simulink model "Kinematic_control_path_tracking"  (R2022b)
settings: Solver=VariableStepAuto  StartTime=0.0  StopTime=T_final*2  RelTol=1e-3
values from neighbouring files (symbols this model uses):
  d = 0.1    [Run_model.m]
  kx = 4    [Run_model.m]
  ky = 4    [Run_model.m]
  R = 1e-5    (= 1e-05)    [Run_model.m]
  Ts = 0.01    [Run_model.m]    (also in imu.m)
  u0 = [0;0]    [Run_model.m]
  z_initial = [theta0;x0;y0]    [Run_model.m]
libraries: simulink x1, sharedTrackingLibrary x1
settings Model: Creator=Abelb  LastModifiedBy=RASLab-Distributed

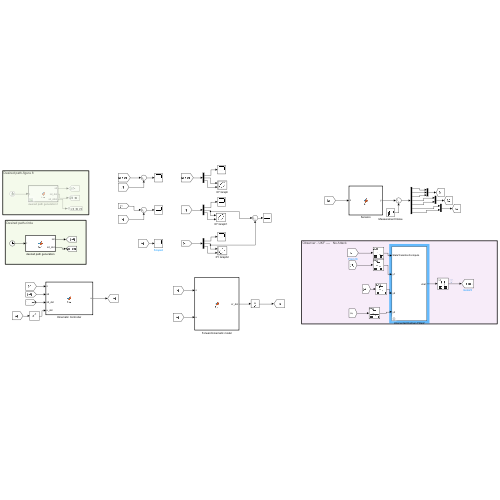
[thumbnail: Simulink's stored preview of the top-level diagram]
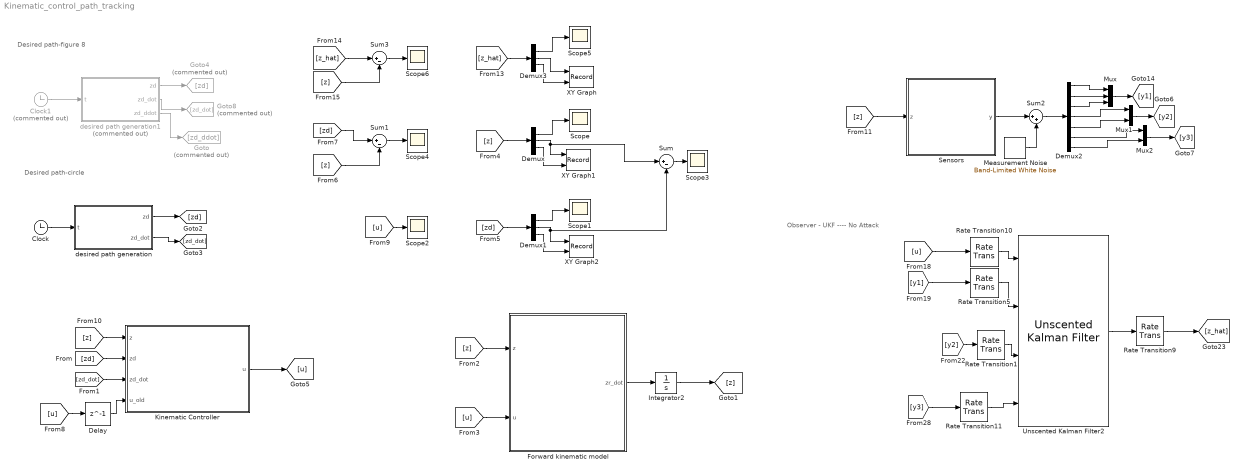
== system Kinematic_control_path_tracking ==
  note: Desired path-circle
  note: Desired path-figure 8
  note: Observer - UKF ---- No Attack
  Clock : Clock
  Clock1 : Clock  Commented=on
  Delay : Delay  DelayLength=1  InitialCondition=u0
  Demux : Demux  Outputs=3
  Demux1 : Demux  Outputs=3
  Demux2 : Demux  Outputs=n_meas
  Demux3 : Demux  Outputs=3
  Forward kinematic model : MATLAB Function  TreatAsAtomicUnit=on
  Goto : Goto  Commented=on  GotoTag=zd_ddot
  Goto4 : Goto  Commented=on  GotoTag=zd
  Goto8 : Goto  Commented=on  GotoTag=zd_dot
  Integrator2 : Integrator  InitialCondition=z_initial
  Kinematic Controller : MATLAB Function  TreatAsAtomicUnit=on
  Measurement Noise : simulink/Sources/Band-Limited White Noise  Cov=R*Ts  Ts=Ts  seed=[23341]
  Mux : Mux  Inputs=3
  Mux1 : Mux  Inputs=2
  Mux2 : Mux  Inputs=2
  Rate Transition1 : RateTransition  InitialCondition=[0 0]  OutPortSampleTime=Ts
  Rate Transition10 : RateTransition  InitialCondition=[0 0]  OutPortSampleTime=Ts
  Rate Transition11 : RateTransition  InitialCondition=[0 0]  OutPortSampleTime=Ts
  Rate Transition5 : RateTransition  InitialCondition=[0 0 0]  OutPortSampleTime=Ts
  Rate Transition9 : RateTransition  Integrity=off  InitialCondition=1.6  OutPortSampleTime=0
  Scope{,1..6} (7 alike) : Scope
  Sensors : MATLAB Function  TreatAsAtomicUnit=on
  Sum : Sum  Inputs=|+-
  Sum1 : Sum  Inputs=|+-
  Sum2 : Sum  Inputs=|++
  Sum3 : Sum  Inputs=|+-
  Unscented Kalman Filter2 : sharedTrackingLibrary/Unscented Kalman Filter  StateTransitionFcn=Dynamicfcn  HasAdditiveProcessNoise=Additive  ProcessNoise=diag([1 1 1])  HasTimeVaryingProcessNoise=off  HasStateTransitionFcnExtraArgument=1  InitialState=z_hat0  InitialStateCovariance=0.1  Alpha=1e-2  Beta=2  Kappa=0  MeasurementFcn1=imu  HasMeasurementEnablePort1=off  HasAdditiveMeasurementNoise1=Additive  MeasurementNoise1=diag([R R R])  HasTimeVaryingMeasurementNoise1=off  HasMeasurementFcnExtraArgument1=0  HasMeasurementWrapping1=off  MeasurementFcn2=encoder  HasMeasurementEnablePort2=off  HasAdditiveMeasurementNoise2=Additive  MeasurementNoise2=diag([R R])  HasTimeVaryingMeasurementNoise2=off  HasMeasurementFcnExtraArgument2=0  HasMeasurementWrapping2=off  MeasurementFcn3=gps  HasMeasurementEnablePort3=off  HasAdditiveMeasurementNoise3=Additive  MeasurementNoise3=diag([R R])  HasTimeVaryingMeasurementNoise3=off  HasMeasurementFcnExtraArgument3=0  HasMeasurementWrapping3=off  MeasurementFcn4=mfcn3  HasMeasurementEnablePort4=off  HasAdditiveMeasurementNoise4=Additive  MeasurementNoise4=R  HasTimeVaryingMeasurementNoise4=off  HasMeasurementFcnExtraArgument4=0  HasMeasurementWrapping4=off  MeasurementFcn5=myMeasurementFcn  HasMeasurementEnablePort5=off  HasAdditiveMeasurementNoise5=Additive  MeasurementNoise5=1  HasTimeVaryingMeasurementNoise5=off  HasMeasurementFcnExtraArgument5=0  HasMeasurementWrapping5=off  EnableMultirate=off  StateTransitionFcnSampleTime=1  MeasurementFcn1SampleTime=1  MeasurementFcn2SampleTime=1  MeasurementFcn3SampleTime=1  MeasurementFcn4SampleTime=1  MeasurementFcn5SampleTime=1  UseCurrentEstimator=off  OutputStateCovariance=off  DataType=double  SampleTime=Ts  NumberOfMeasurements=3
  XY Graph : Record  FileSettingsInternal="{\"entries\":[{\"content\":{\"excelSettings\":{\"content\":{},\"type\":\"Streamout.ExcelSettings\"}},\"type\":\"Streamout.FileSettingStorage\",\"uuid\":\"53b03b39-55e0-4fa9-afe4-2bd9ebb48c30\"}],\"packageUris\":[\"http://schema.mathworks.com/mf0/streamout_blocks/R2020a\"],\"version\":\"1.0\"}"  Layout=[1 1]  SignalsInternal="{\"entries\":[{\"content\":{\"signals\":[{\"content\":{\"blockPath\":[\"Kinematic_control_path_tracking/XY Graph\"],\"channel\":[],\"dimensions\":[1],\"domain\":\"Kinematic_control_path_tracking/XY Graph\",\"lineColor\":\"#a2142f\",\"plots\":[1],\"port\":1,\"sid\":[\"\"],\"signalID\":23982,\"signalName\":\"Demux3:2\"},\"type\":\"RecordBlkView.Signal\",\"uuid\":\"5156a42c-5bae-4aca-bacc-39f4cef39f7f\"},{\"content\":{\"blockPath\":[\"Kinematic_control_path_tracking/XY Graph\"],\"channel\":[],\"dimensions\":[1],\"domain\":\"Kinematic_control_path_tracking/XY Graph\",\"lineColor\":\"#139fff\",\"plots\":[1],\"port\":2,\"sid\":[\"\"],\"signalID\":23986,\"signalName\":\"Demux3:3\"},\"type\":\"RecordBlkView.Signal\",\"uuid\":\"2cf1826c-70a3-4cdb-a73e-eee623f68542\"}]},\"type\":\"RecordBlkView.InputSignals\",\"uuid\":\"c4e639f7-235e-4a76-b281-eb1d9f92212a\"}],\"packageUris\":[\"http://schema.mathworks.com/mf0/streamout_blocks/R2020a\"],\"version\":\"1.0\"}"  VisualizationBindings="{\"xyplotplugin\":{\"info\":[{\"series\":[{\"bindingParametersList\":[{\"parameter\":\"X-Axis\",\"signalID\":23982,\"signalName\":\"Demux3:2\"},{\"parameter\":\"Y-Axis\",\"signalID\":23986,\"signalName\":\"Demux3:3\"}],\"seriesID\":42700}],\"subplotID\":1}]}}"  CompatibilityTag=XY
  XY Graph1 : Record  FileSettingsInternal="{\"entries\":[{\"content\":{\"excelSettings\":{\"content\":{},\"type\":\"Streamout.ExcelSettings\"}},\"type\":\"Streamout.FileSettingStorage\",\"uuid\":\"22695cf6-89d7-43ca-b8cc-e55b69a454ec\"}],\"packageUris\":[\"http://schema.mathworks.com/mf0/streamout_blocks/R2020a\"],\"version\":\"1.0\"}"  Layout=[1 1]  SignalsInternal="{\"entries\":[{\"content\":{\"signals\":[{\"content\":{\"blockPath\":[\"Kinematic_control_path_tracking/XY Graph1\"],\"channel\":[],\"dimensions\":[1],\"domain\":\"Kinematic_control_path_tracking/XY Graph1\",\"lineColor\":\"#a2142f\",\"plots\":[1],\"port\":1,\"sid\":[\"\"],\"signalID\":23990,\"signalName\":\"Demux:2\"},\"type\":\"RecordBlkView.Signal\",\"uuid\":\"5f30c967-a085-4e3c-978a-3d45b454423d\"},{\"content\":{\"blockPath\":[\"Kinematic_control_path_tracking/XY Graph1\"],\"channel\":[],\"dimensions\":[1],\"domain\":\"Kinematic_control_path_tracking/XY Graph1\",\"lineColor\":\"#139fff\",\"plots\":[1],\"port\":2,\"sid\":[\"\"],\"signalID\":23994,\"signalName\":\"Demux:3\"},\"type\":\"RecordBlkView.Signal\",\"uuid\":\"e37d4cd6-5af5-4e48-88eb-1684f785dfd2\"}]},\"type\":\"RecordBlkView.InputSignals\",\"uuid\":\"b7753eae-dfa1-472a-a4ee-c8d1f4983262\"}],\"packageUris\":[\"http://schema.mathworks.com/mf0/streamout_blocks/R2020a\"],\"version\":\"1.0\"}"  VisualizationBindings="{\"xyplotplugin\":{\"info\":[{\"series\":[{\"bindingParametersList\":[{\"parameter\":\"X-Axis\",\"signalID\":23990,\"signalName\":\"Demux:2\"},{\"parameter\":\"Y-Axis\",\"signalID\":23994,\"signalName\":\"Demux:3\"}],\"seriesID\":7810}],\"subplotID\":1}]}}"  CompatibilityTag=XY
  XY Graph2 : Record  FileSettingsInternal="{\"entries\":[{\"content\":{\"excelSettings\":{\"content\":{},\"type\":\"Streamout.ExcelSettings\"}},\"type\":\"Streamout.FileSettingStorage\",\"uuid\":\"eace55e5-3c6d-4366-b246-c90901abd758\"}],\"packageUris\":[\"http://schema.mathworks.com/mf0/streamout_blocks/R2020a\"],\"version\":\"1.0\"}"  Layout=[1 1]  SignalsInternal="{\"entries\":[{\"content\":{\"signals\":[{\"content\":{\"blockPath\":[\"Kinematic_control_path_tracking/XY Graph2\"],\"channel\":[],\"dimensions\":[1],\"domain\":\"Kinematic_control_path_tracking/XY Graph2\",\"lineColor\":\"#a2142f\",\"plots\":[1],\"port\":1,\"sid\":[\"\"],\"signalID\":23998,\"signalName\":\"Demux1:2\"},\"type\":\"RecordBlkView.Signal\",\"uuid\":\"c09d6a8b-b75d-4225-bd49-b55b8471079b\"},{\"content\":{\"blockPath\":[\"Kinematic_control_path_tracking/XY Graph2\"],\"channel\":[],\"dimensions\":[1],\"domain\":\"Kinematic_control_path_tracking/XY Graph2\",\"lineColor\":\"#139fff\",\"plots\":[1],\"port\":2,\"sid\":[\"\"],\"signalID\":24002,\"signalName\":\"Demux1:3\"},\"type\":\"RecordBlkView.Signal\",\"uuid\":\"1f0564bc-c8d1-4d71-ab9b-9d1cb6ef22b8\"}]},\"type\":\"RecordBlkView.InputSignals\",\"uuid\":\"f5b7b8dd-13dd-4d16-8a9c-72a61d8133b0\"}],\"packageUris\":[\"http://schema.mathworks.com/mf0/streamout_blocks/R2020a\"],\"version\":\"1.0\"}"  VisualizationBindings="{\"xyplotplugin\":{\"info\":[{\"series\":[{\"bindingParametersList\":[{\"parameter\":\"X-Axis\",\"signalID\":23998,\"signalName\":\"Demux1:2\"},{\"parameter\":\"Y-Axis\",\"signalID\":24002,\"signalName\":\"Demux1:3\"}],\"seriesID\":9465}],\"subplotID\":1}]}}"  CompatibilityTag=XY
  desired path generation : MATLAB Function  TreatAsAtomicUnit=on
  desired path generation1 : MATLAB Function  Commented=on  TreatAsAtomicUnit=on
  wires:
  Forward kinematic model/1(zr_dot) -> Integrator2/1
  desired path generation1/3(zd_ddot) -> Goto/1
  Clock1/1 -> desired path generation1/1(t)
  desired path generation1/2(zd_dot) -> Goto8/1
  desired path generation1/1(zd) -> Goto4/1
  desired path generation/2(zd_dot) -> [zd_dot]
  desired path generation/1(zd) -> [zd]
  Clock/1 -> desired path generation/1(t)
  [zd] -> Kinematic Controller/2(zd)
  [zd_dot] -> Kinematic Controller/3(zd_dot)
  Integrator2/1 -> [z]
  [z] -> Forward kinematic model/1(z)
  [z] -> Demux/1
  Demux/1 -> Scope/1
  Demux/2 -> XY Graph1/1, Sum/1
  Demux/3 -> XY Graph1/2
  Demux1/2 -> XY Graph2/1, Sum/2
  Demux1/3 -> XY Graph2/2
  [zd] -> Demux1/1
  Demux1/1 -> Scope1/1
  Sum/1 -> Scope3/1
  Delay/1 -> Kinematic Controller/4(u_old)
  Kinematic Controller/1(u) -> [u]
  [zd] -> Sum1/1
  [z] -> Sum1/2
  Sum1/1 -> Scope4/1
  [y1] -> Rate Transition5/1
  Unscented Kalman Filter2/1 -> Rate Transition9/1
  [y3] -> Rate Transition11/1
  Rate Transition9/1 -> [z_hat]
  Rate Transition10/1 -> Unscented Kalman Filter2/1
  Rate Transition11/1 -> Unscented Kalman Filter2/4
  [y2] -> Rate Transition1/1
  Rate Transition1/1 -> Unscented Kalman Filter2/3
  Rate Transition5/1 -> Unscented Kalman Filter2/2
  [u] -> Rate Transition10/1
  [u] -> Delay/1
  [u] -> Scope2/1
  [z] -> Sensors/1(z)
  Sensors/1(y) -> Sum2/1
  Measurement Noise/1 -> Sum2/2
  Sum2/1 -> Demux2/1
  Demux2/1 -> Mux/1
  Demux2/2 -> Mux/2
  Mux/1 -> [y1]
  Mux1/1 -> [y2]
  Mux2/1 -> [y3]
  Demux3/2 -> XY Graph/1
  Demux3/1 -> Scope5/1
  Demux3/3 -> XY Graph/2
  [z_hat] -> Demux3/1
  [z] -> Sum3/2
  [z_hat] -> Sum3/1
  Sum3/1 -> Scope6/1
  [u] -> Forward kinematic model/2(u)
  Demux2/7 -> Mux2/2
  Demux2/6 -> Mux2/1
  Demux2/5 -> Mux1/2
  Demux2/4 -> Mux1/1
  Demux2/3 -> Mux/3
  [z] -> Kinematic Controller/1(z)

== matlab function Kinematic_control_path_tracking/desired path generation1 ==
  data: t input; zd output; zd_dot output; zd_ddot output
function [zd,zd_dot,zd_ddot] = fcn(t)

t = t/50;

a=1;
x = a*cos(t)/(1+sin(t)^2);
y = a*sin(t)*cos(t)/(1+sin(t)^2);
% unit circle (radius = 1; origin: (0,0))
zd = [atan(y./x);              % theta
      a*cos(t)/(1+sin(t)^2);         % x
      a*sin(t)*cos(t)/(1+sin(t)^2)];        % y

zd_dot = [ 0;
          -a*sin(t)*(cos(t)^2+2)/(1+sin(t)^2)^2;
          (a*cos(t)^2-2*a*sin(t)^2)/(1+sin(t)^2)^2];

z1 = (a*sin(t)^2*cos(t)^3-11*a*cos(t)^3+8*a*cos(t))/(1+sin(t)^2)^3;
z2 = -2*a*sin(t)*cos(t)*(3+2*cos(t)^2-sin(t)^2)/(1+sin(t)^2)^3;
zd_ddot = [z1;
           z2];

== matlab function Kinematic_control_path_tracking/Kinematic Controller ==
  data: z input; u output; zd input; zd_dot input; u_old input; d parameter; kx parameter; ky parameter
function u = fcn(z,zd,zd_dot,u_old,d, kx, ky)

%% unpacking inputs
theta = z(1);
x = z(2);
y = z(3);
xd = zd(2);
yd = zd(3);
xd_dot = zd_dot(2);
yd_dot = zd_dot(3);

v_old = u_old(1);
omega_old = u_old(2);


%% controller
K1 = [cos(theta) sin(theta);
     -sin(theta)/d cos(theta)/d];
K2 = [xd_dot + kx*sin( atan( kx*(xd-x) ) );
      yd_dot + ky*sin( atan( ky*(yd-y) ) )];
u = K1*K2;



%% rate constraint (physics)
v = u(1);
omega = u(2);

% v = min(max(max(min(v_old+0.1,v),v_old-0.1),-0.5),0.5);
% omega =  min(max(max(min(omega_old+0.25,omega),omega_old-0.25),-1.75),1.75);

%% packing output
u = [v;
     omega];

== matlab function Kinematic_control_path_tracking/Sensors ==
  data: z input; y output
function y = fcn(z)

coder.extrinsic('imu');
coder.extrinsic('encoder');
coder.extrinsic('gps');

y1 = zeros(3,1);
y2 = zeros(2,1);
y3 = zeros(2,1);

y1(:) = imu(z);
y2(:) = encoder(z);
y3(:) = gps(z);

y = [y1;
     y2;
     y3];

== matlab function Kinematic_control_path_tracking/Forward kinematic model ==
  data: z input; u input; zr_dot output; d parameter
function zr_dot = fcn(z,u,d)

%% unpacking the state vectors
theta=z(1);

%% unpacking the intput
v=u(1);
omega=u(2);

%% ODE
theta_dot=omega;
x_dot=v*cos(theta)-d*omega*sin(theta);
y_dot=v*sin(theta)+d*omega*cos(theta);
% phir_dot = (v+omega)/r;
% phil_dot = (v-omega)/r;


%% packing the output
zr_dot=[theta_dot;x_dot;y_dot];

== matlab function Kinematic_control_path_tracking/desired path generation ==
  data: t input; zd output; zd_dot output
function [zd,zd_dot] = fcn(t)

 t = t/50;


% unit circle (radius = 1; origin: (0,0))
zd = [t;
      sin(2*t);         % x
      1-cos(2*t)];        % y

zd_dot = [1;
          2*cos(2*t);
          2*sin(2*t)];
